simulink model "test_increase_button_earlyrelease"  (R2022b)
settings: Solver=FixedStepAuto  StartTime=0.0  StopTime=240  FixedStep=0.1  RelTol=1e-3
settings Model: Creator=cristian  LastModifiedBy=cristian
settings ConfigComp: CovEnable=on  RecordCoverage=on  CovModelRefEnable=on

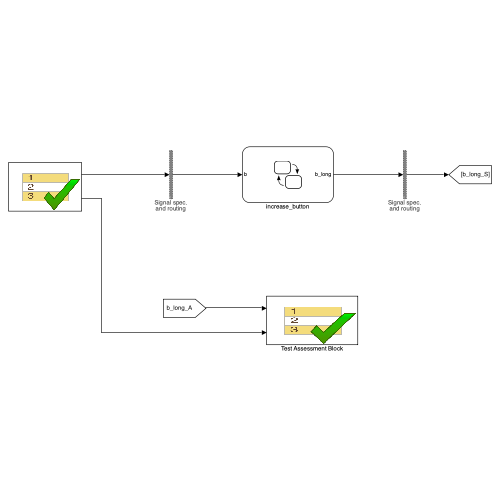
[thumbnail: Simulink's stored preview of the top-level diagram]
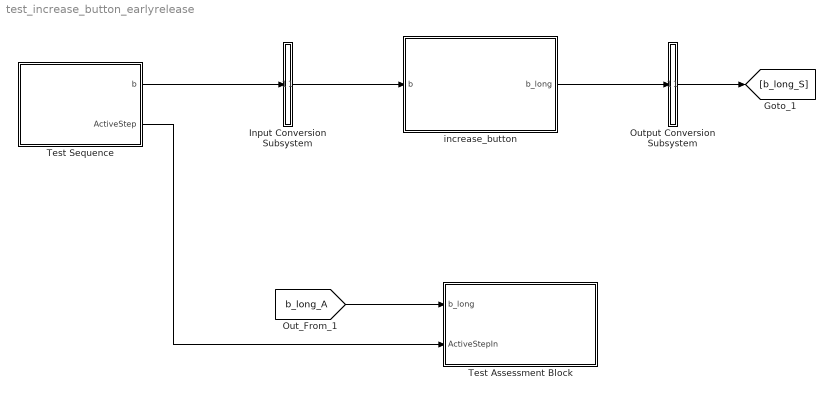
== system test_increase_button_earlyrelease ==
  Input Conversion Subsystem : Subsystem  Tag=__SLT_ICS__  Description=|
      | Signal spec.
      | and routing
      settings: AttributesFormatString=%<Description>
  Output Conversion Subsystem : Subsystem  Tag=__SLT_OCS__  Description=|
      | Signal spec.
      | and routing
      settings: AttributesFormatString=%<Description>
  Test Assessment Block : Test Sequence  Tag=__SLT_ASMT__  TreatAsAtomicUnit=on
  Test Sequence : Test Sequence  TreatAsAtomicUnit=on
  increase_button : Stateflow chart  TreatAsAtomicUnit=on
  wires:
  Test Sequence/1(b) -> Input Conversion Subsystem/1(Inport_1)
  Output Conversion Subsystem/1(Outport_1) -> [b_long_S]
  Input Conversion Subsystem/1(Outport_1) -> increase_button/1(b)
  increase_button/1(b_long) -> Output Conversion Subsystem/1(Inport_1)
  Test Sequence/2(ActiveStep) -> Test Assessment Block/2(ActiveStepIn)
  [b_long_A] -> Test Assessment Block/1(b_long)

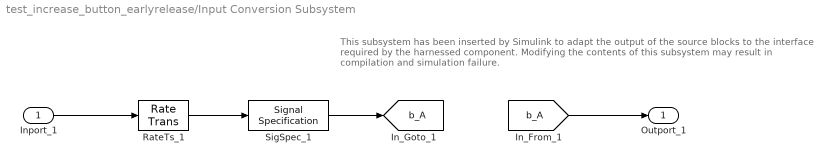
== system test_increase_button_earlyrelease/Input Conversion Subsystem ==
  note: This subsystem has been inserted by Simulink to adapt the output of the source blocks to the interface required by the harnessed component.
      |  Modifying the contents of this subsystem may result in compilation and simulation failure.
  Inport_1 : Inport
  RateTs_1 : RateTransition  OutPortSampleTime=[-1, 0]
  SigSpec_1 : SignalSpecification  OutDataTypeStr=boolean  Dimensions=[1]  SampleTime=[-1, 0]
  Outport_1 : Outport
  tag scope: b_A=global
  wires:
  [b_A] -> Outport_1/1
  SigSpec_1/1 -> [b_A]
  RateTs_1/1 -> SigSpec_1/1
  Inport_1/1 -> RateTs_1/1

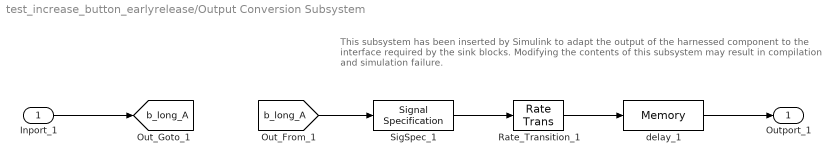
== system test_increase_button_earlyrelease/Output Conversion Subsystem ==
  note: This subsystem has been inserted by Simulink to adapt the output of the harnessed component to the interface required by the sink blocks.
      |  Modifying the contents of this subsystem may result in compilation and simulation failure.
  Inport_1 : Inport
  Rate_Transition_1 : RateTransition  OutPortSampleTimeOpt=Inherit
  SigSpec_1 : SignalSpecification  OutDataTypeStr=boolean  Dimensions=[1]
  delay_1 : Memory
  Outport_1 : Outport
  tag scope: b_long_A=global
  wires:
  Inport_1/1 -> [b_long_A]
  [b_long_A] -> SigSpec_1/1
  SigSpec_1/1 -> Rate_Transition_1/1
  Rate_Transition_1/1 -> delay_1/1
  delay_1/1 -> Outport_1/1

== stateflow chart test_increase_button_earlyrelease/Test Assessment Block ==
  state EarlyRelease
    state Run
      settings: description=Esecuzione test
      state Verify_ER_Init
        verify(b_long == 1);
        settings: description=Inizialmente il pulsante non è premuto.
      state Verify_ER_ButtonPressed
        verify(b_long == 1);
        settings: description=Viene premuto il pulsante, ma non per un tempo sufficientemente lungo da richiedere un cambio potenza.
      state Verify_ER_ButtonReleased
        verify(b_long == 1);
        settings: description=Quando il pulsante viene rilasciato (prima di un secondo, perché abbiamo scelto 0.5), la pressione lunga non viene rilevata.
      state step_1_2
      Run -> (junction 234)
      (default) -> (junction 234)
      (junction 234) -> (junction 235) [order 1] : [ActiveStepIn == ActiveStepEnumH1.ER_Init
          | ]
      (junction 235) -> Verify_ER_Init [order 1] : [~in(EarlyRelease.Run.Verify_ER_Init)]
      (junction 234) -> (junction 243) [order 2]
      (junction 235) -> (junction 238) [order 2]
      (junction 243) -> (junction 244) [order 1] : [ActiveStepIn == ActiveStepEnumH1.ER_ButtonPressed
          | ]
      (junction 244) -> Verify_ER_ButtonPressed [order 1] : [~in(EarlyRelease.Run.Verify_ER_ButtonPressed)]
      (junction 243) -> (junction 258) [order 2]
      (junction 244) -> (junction 247) [order 2]
      (junction 258) -> (junction 259) [order 1] : [ActiveStepIn == ActiveStepEnumH1.ER_ButtonReleased
          | ]
      (junction 259) -> Verify_ER_ButtonReleased [order 1] : [~in(EarlyRelease.Run.Verify_ER_ButtonReleased)]
      (junction 258) -> (junction 266) [order 2]
      (junction 259) -> (junction 262) [order 2]
      (junction 266) -> (junction 267)
      (junction 267) -> step_1_2 [order 1] : [~in(EarlyRelease.Run.step_1_2)]
      (junction 267) -> (junction 270) [order 2]
    (default) -> Run
  (default) -> EarlyRelease : {assert(Active_Scenario_Index == 1,'The value of Scenario Parameter ''Active_Scenario_Index'' is not valid. Use the index of the scenario to specify it.')}
  data: b_long input boolean size=[1]; ActiveStepIn input; Active_Scenario_Index parameter =1; sampleTime constant double =str2num(get_param('InductionCooker','FixedStep'))

== stateflow chart test_increase_button_earlyrelease/Test Sequence ==
  settings: updateMethod=DISCRETE  sampleTime=0.1
  state EarlyRelease
    state ER_Init
      %% Initialize data outputs.
      b = true;
      settings: description=|
          | Pulsante non premuto.
          | Il pulsante lavora in logica negata come avviene per il bottone presente sulla scheda.
    state ER_ButtonPressed
      b = false
      settings: description=|
          | Pulsante premuto.
          | Lo stato passa da Wait a Pressed.
          | Consideriamo questo step attivo per meno di 1 secondo (ad esempio mezzo secondo).
    state ER_ButtonReleased
      b = true
      settings: description=|
          | Pulsante rilasciato dopo mezzo secondo.
          | Lo stato passa da Pressed a Wait.
          | Ci aspettiamo che non sia stata rilevata la richiesta di aumento della potenza.
    (default) -> ER_Init
    ER_Init -> ER_ButtonPressed : [
        | true
        | ]
    ER_ButtonPressed -> ER_ButtonReleased : [
        | after(0.5,sec)
        | ]
  (default) -> EarlyRelease : {assert(Active_Scenario_Index == 1,'The value of Scenario Parameter ''Active_Scenario_Index'' is not valid. Use the index of the scenario to specify it.')}
  data: b output boolean size=[1]; ActiveStep output Enum: ActiveStepEnumH1; sampleTime constant double =str2num(get_param('InductionCooker','FixedStep')); Active_Scenario_Index parameter =1

== stateflow chart test_increase_button_earlyrelease/increase_button ==
  note: Bottone a livelli, la pressione per un numero di secondi pari a DURATION permette di avere un uscita alta in maniera istantanea.
      | Per avere in output un valore PRESSED, è necessare lasciare il bottone e premere tra un output e l'altro.
  state Wait
    en: b_long = RELEASED
  state Pressed
    en: b_long = RELEASED;
    on after(DURATION,sec): b_long = PRESSED
  state LongPressed
    en: b_long = RELEASED
  (default) -> Wait
  Wait -> Pressed : [b == PRESSED]
  Pressed -> Wait [order 1] : [b == RELEASED]
  LongPressed -> Wait : [b == RELEASED]
  Pressed -> LongPressed [order 2] : [b_long == PRESSED && b == PRESSED]
  data: b_long output boolean size=1; PRESSED constant boolean size=1 =0; RELEASED constant boolean size=1 =1; b input boolean size=1; DURATION constant double size=1 =1
